simulink model "AEB_Main_System"  (R2025b)
settings: Solver=FixedStepDiscrete  StartTime=0.0  StopTime=15.0  FixedStep=Ts  RelTol=1e-3
undefined symbols (not defined in the file): a_max_brake, DiscIntNeverNeededParam, v0_ego
libraries: simulink x2
settings Model: Creator=Hari  LastModifiedBy=Hari

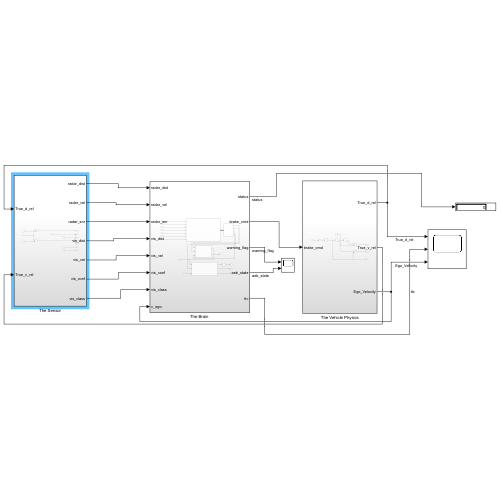
[thumbnail: Simulink's stored preview of the top-level diagram]
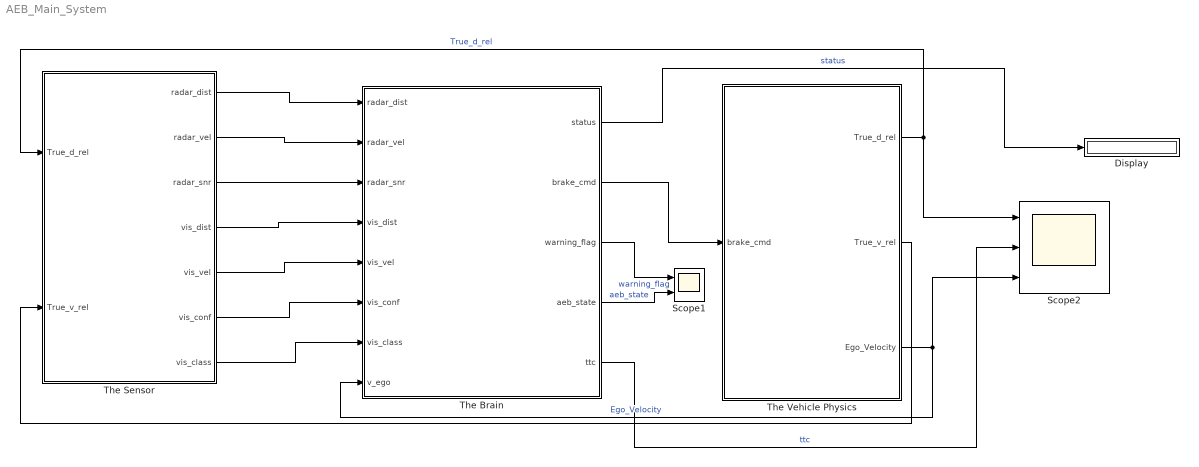
== system AEB_Main_System ==
  Display : Display
  Scope1 : Scope  NumInputPorts=2
      settings: ActiveDisplayYMinimum=-0.41434945554892644  ActiveDisplayYMaximum=2.4797130444510747
  Scope2 : Scope  NumInputPorts=3
      settings: ActiveDisplayYMinimum=-18.191257915372553  ActiveDisplayYMaximum=212.53330153884539  DataLoggingVariableName=ScopeData2
  "The Brain " : Subsystem
  The Sensor : Subsystem
  The Vehicle Physics : Subsystem
  wires:
  "The Brain "/2(brake_cmd) -> The Vehicle Physics/1(brake_cmd)
  The Sensor/1(radar_dist) -> "The Brain "/1(radar_dist)
  The Sensor/2(radar_vel) -> "The Brain "/2(radar_vel)
  The Sensor/3(radar_snr) -> "The Brain "/3(radar_snr)
  The Sensor/4(vis_dist) -> "The Brain "/4(vis_dist)
  The Sensor/5(vis_vel) -> "The Brain "/5(vis_vel)
  The Sensor/6(vis_conf) -> "The Brain "/6(vis_conf)
  The Sensor/7(vis_class) -> "The Brain "/7(vis_class)
  The Vehicle Physics/3(Ego_Velocity) -> Scope2/3, "The Brain "/8(v_ego)  "Ego_Velocity"
  The Vehicle Physics/1(True_d_rel) -> Scope2/1, The Sensor/1(True_d_rel)  "True_d_rel"
  The Vehicle Physics/2(True_v_rel) -> The Sensor/2(True_v_rel)
  "The Brain "/4(aeb_state) -> Scope1/2  "aeb_state"
  "The Brain "/1(status) -> Display/1  "status"
  "The Brain "/3(warning_flag) -> Scope1/1  "warning_flag"
  "The Brain "/5(ttc) -> Scope2/2  "ttc"

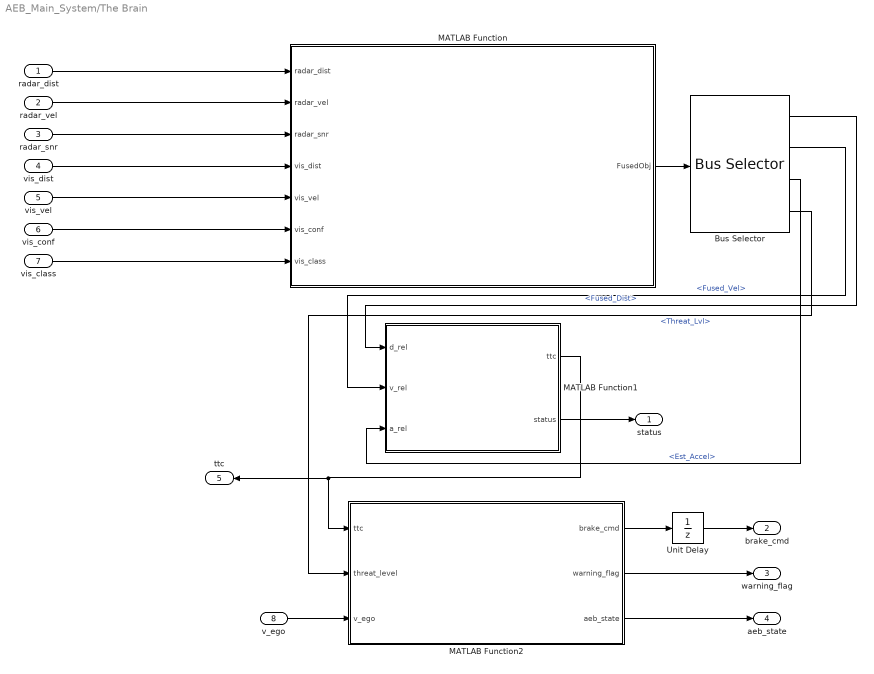
== system AEB_Main_System/The Brain  ==
  radar_dist : Inport
  radar_vel : Inport  Port=2
  radar_snr : Inport  Port=3
  vis_dist : Inport  Port=4
  vis_vel : Inport  Port=5
  vis_conf : Inport  Port=6
  vis_class : Inport  Port=7
  v_ego : Inport  Port=8
  Bus Selector : BusSelector  OutputSignals=Fused_Dist,Fused_Vel,Est_Accel,Threat_Lvl
  MATLAB Function : MATLAB Function  TreatAsAtomicUnit=on
  MATLAB Function1 : MATLAB Function  TreatAsAtomicUnit=on
  MATLAB Function2 : MATLAB Function  TreatAsAtomicUnit=on
  Unit Delay : UnitDelay  SampleTime=-1  HasFrameUpgradeWarning=on
  status : Outport
  brake_cmd : Outport  Port=2
  warning_flag : Outport  Port=3
  aeb_state : Outport  Port=4
  ttc : Outport  Port=5
  wires:
  radar_dist/1 -> MATLAB Function/1(radar_dist)
  radar_vel/1 -> MATLAB Function/2(radar_vel)
  radar_snr/1 -> MATLAB Function/3(radar_snr)
  vis_dist/1 -> MATLAB Function/4(vis_dist)
  vis_vel/1 -> MATLAB Function/5(vis_vel)
  vis_conf/1 -> MATLAB Function/6(vis_conf)
  vis_class/1 -> MATLAB Function/7(vis_class)
  MATLAB Function1/2(status) -> status/1
  MATLAB Function1/1(ttc) -> ttc/1, MATLAB Function2/1(ttc)
  v_ego/1 -> MATLAB Function2/3(v_ego)
  MATLAB Function2/2(warning_flag) -> warning_flag/1
  MATLAB Function2/3(aeb_state) -> aeb_state/1
  MATLAB Function/1(FusedObj) -> Bus Selector/1
  Bus Selector/1 -> MATLAB Function1/1(d_rel)  "<Fused_Dist>"
  Bus Selector/2 -> MATLAB Function1/2(v_rel)  "<Fused_Vel>"
  Bus Selector/4 -> MATLAB Function2/2(threat_level)  "<Threat_Lvl>"
  Bus Selector/3 -> MATLAB Function1/3(a_rel)  "<Est_Accel>"
  MATLAB Function2/1(brake_cmd) -> Unit Delay/1
  Unit Delay/1 -> brake_cmd/1

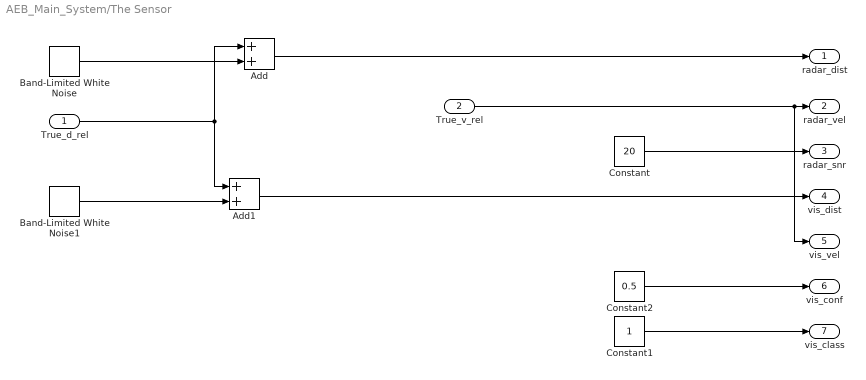
== system AEB_Main_System/The Sensor ==
  True_d_rel : Inport
  True_v_rel : Inport  Port=2
  Add : Sum
  Add1 : Sum
  Band-Limited White Noise : simulink/Sources/Band-Limited White Noise  Cov=[0.5]  Ts=0.1  seed=[23341]
  Band-Limited White Noise1 : simulink/Sources/Band-Limited White Noise  Cov=[1.5]  Ts=0.1  seed=[23341]
  Constant : Constant  Value=20
  Constant1 : Constant
  Constant2 : Constant  Value=0.5
  radar_dist : Outport
  radar_vel : Outport  Port=2
  radar_snr : Outport  Port=3
  vis_dist : Outport  Port=4
  vis_vel : Outport  Port=5
  vis_conf : Outport  Port=6
  vis_class : Outport  Port=7
  wires:
  True_d_rel/1 -> Add1/1, Add/1
  Band-Limited White Noise/1 -> Add/2
  Add/1 -> radar_dist/1
  Band-Limited White Noise1/1 -> Add1/2
  Add1/1 -> vis_dist/1
  True_v_rel/1 -> vis_vel/1, radar_vel/1
  Constant/1 -> radar_snr/1
  Constant2/1 -> vis_conf/1
  Constant1/1 -> vis_class/1

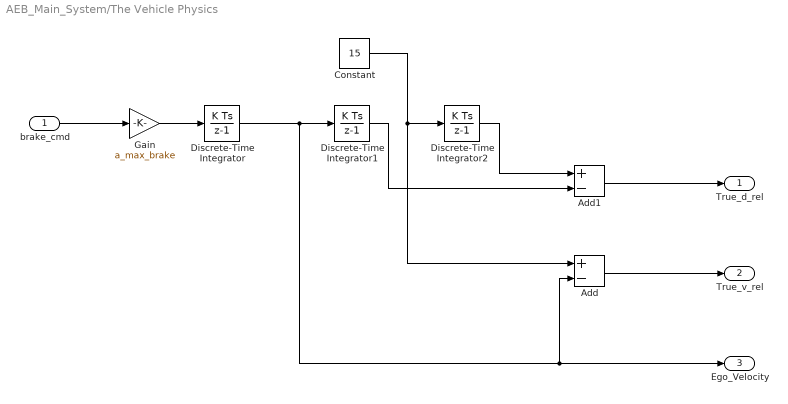
== system AEB_Main_System/The Vehicle Physics ==
  brake_cmd : Inport
  Add : Sum  Inputs=+-
  Add1 : Sum  Inputs=+-
  Constant : Constant  Value=15
  Discrete-Time Integrator : DiscreteIntegrator  InitialCondition=v0_ego  SampleTime=-1  ICPrevOutput=DiscIntNeverNeededParam  ICPrevScaledInput=DiscIntNeverNeededParam
  Discrete-Time Integrator1 : DiscreteIntegrator  SampleTime=-1  ICPrevOutput=DiscIntNeverNeededParam  ICPrevScaledInput=DiscIntNeverNeededParam
  Discrete-Time Integrator2 : DiscreteIntegrator  InitialCondition=70  SampleTime=-1  ICPrevOutput=DiscIntNeverNeededParam  ICPrevScaledInput=DiscIntNeverNeededParam
  Gain : Gain  Gain=a_max_brake
  True_d_rel : Outport
  True_v_rel : Outport  Port=2
  Ego_Velocity : Outport  Port=3
  wires:
  brake_cmd/1 -> Gain/1
  Discrete-Time Integrator1/1 -> Add1/2
  Discrete-Time Integrator/1 -> Add/2, Ego_Velocity/1, Discrete-Time Integrator1/1
  Gain/1 -> Discrete-Time Integrator/1
  Constant/1 -> Add/1, Discrete-Time Integrator2/1
  Discrete-Time Integrator2/1 -> Add1/1
  Add1/1 -> True_d_rel/1
  Add/1 -> True_v_rel/1

== matlab function AEB_Main_System/The Brain /MATLAB Function1 ==
  data: d_rel input; ttc output; v_rel input; a_rel input; status output
function [ttc, status] = calc_ttc(d_rel, v_rel, a_rel)
    % SIXXIS Advanced: 2nd-Order Kinematic Prediction Engine
    
    ttc = 5.0; 
    status = 0;

    % Relative velocity check: Is collision possible?
    if v_rel >= 0 && a_rel >= 0
        return; 
    end

    % Solve for t in: 0.5*a*t^2 + v*t + d = 0
    discriminant = (v_rel^2) - (2 * a_rel * d_rel);

    if discriminant >= 0
        if abs(a_rel) > 0.05
            % Using Quadratic Formula
            t1 = (-v_rel + sqrt(discriminant)) / a_rel;
            t2 = (-v_rel - sqrt(discriminant)) / a_rel;
            
            roots_found = [t1, t2];
            valid_roots = roots_found(roots_found > 0);
            if ~isempty(valid_roots)
                ttc = min(valid_roots);
                status = 1;
            end
        else
            % Fallback to 1st order linear if acceleration is near zero
            if v_rel < 0
                ttc = -d_rel / v_rel;
                status = 1;
            end
        end
    end
    
    % Clamp TTC values for stability
    if ttc > 5.0 || ttc < 0
        ttc = 5.0;
        status = 0;
    end
end

== matlab function AEB_Main_System/The Brain /MATLAB Function ==
  data: radar_dist input; FusedObj output Bus: Bus_Fused; radar_vel input; radar_snr input; vis_dist input; vis_vel input; vis_conf input; vis_class input
function FusedObj = sensor_weighting_fusion(radar_dist, radar_vel, radar_snr, vis_dist, vis_vel, vis_conf, vis_class)
    % SIXXIS Predict-Fusion: Dynamic Sensor Weighting Logic
    
    dt = 0.01; % Deterministic 10ms Step
    
    persistent prev_vel
    if isempty(prev_vel)
        prev_vel = 0;
    end

    % Logic to weight sensors based on confidence/SNR
    w_radar = 0.5; 
    w_vision = 0.5;

    if vis_conf < 0.4 
        w_radar = 0.9; 
        w_vision = 0.1;
    elseif radar_snr < 10
        w_radar = 0.2; 
        w_vision = 0.8;
    end

    % Calculate Fused Outputs
    FusedObj.Fused_Dist = (radar_dist * w_radar) + (vis_dist * w_vision);
    FusedObj.Fused_Vel  = (radar_vel * w_radar) + (vis_vel * w_vision);
    FusedObj.Est_Accel  = (FusedObj.Fused_Vel - prev_vel) / dt;

    % Threat classification
    FusedObj.Threat_Lvl = uint8(0);
    if FusedObj.Fused_Dist < 100 && vis_class > 0
        FusedObj.Threat_Lvl = uint8(1); 
    end

    prev_vel = FusedObj.Fused_Vel;
end

== matlab function AEB_Main_System/The Brain /MATLAB Function2 ==
  data: ttc input; brake_cmd output; threat_level input; v_ego input; warning_flag output; aeb_state output
function [brake_cmd, warning_flag, aeb_state] = aeb_state_machine(ttc, threat_level, v_ego)
    persistent current_state startup_ticks
    if isempty(current_state)
        current_state = 0; 
        startup_ticks = 0; % Counter to ignore initialization spikes
    end

    % 1. Warm-up Period: Ignore first 10 ticks (0.1s) to let sensors stabilize
    if startup_ticks < 10
        startup_ticks = startup_ticks + 1;
        brake_cmd = 0; warning_flag = false; aeb_state = 0;
        return;
    end

    % 2. Thresholds (Same as before)
    TTC_EMERGENCY = 0.8;
    TTC_PARTIAL = 1.2;
    TTC_WARN = 2.0;

    % 3. Latching Logic (The Hysteresis we discussed)
    if current_state == 3 && v_ego > 0.1
        current_state = 3; % Stay in emergency till stopped
    elseif threat_level == 0 || v_ego < 0.1
        current_state = 0; 
    else
        if ttc > 0 && ttc <= TTC_EMERGENCY
            current_state = 3; 
        elseif ttc <= TTC_PARTIAL && current_state < 3
            current_state = 2;
        elseif ttc <= TTC_WARN && current_state < 2
            current_state = 1;
        end
    end

    % 4. Actuation
    switch current_state
        case 3; brake_cmd = 1.0; warning_flag = true;
        case 2; brake_cmd = 0.5; warning_flag = true;
        case 1; brake_cmd = 0.0; warning_flag = true;
        otherwise; brake_cmd = 0.0; warning_flag = false;
    end
    aeb_state = current_state;
end
